simulink model "etp_model"  (R2026a)
settings: Solver=ode15s  StartTime=0  StopTime=1800  MaxStep=0.5  RelTol=1e-6  AbsTol=1e-9
InitFcn:
  | if ~evalin('base','exist(''Qext_ts'',''var'')'),
  |   p_ = evalin('base','p');
  |   Qext_ts = timeseries(p_.Qext_profile.value, p_.Qext_profile.time);
  |   assignin('base','Qext_ts',Qext_ts);
  | end
settings Model: Creator=fsk  LastModifiedBy=fsk

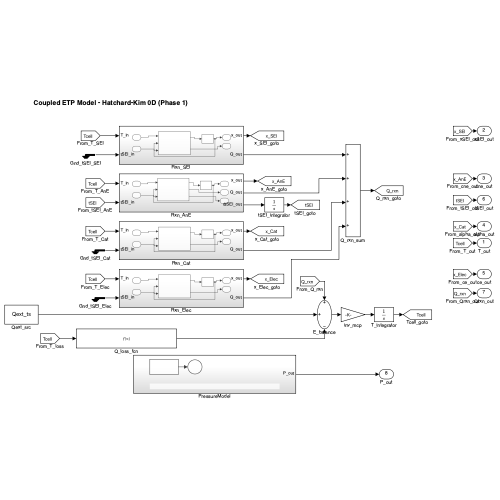
[thumbnail: Simulink's stored preview of the top-level diagram]
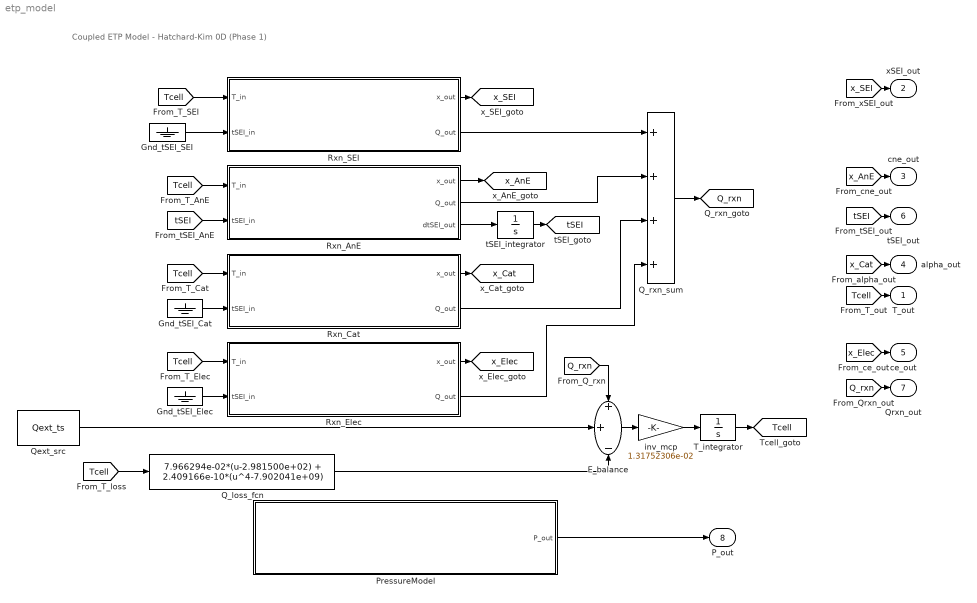
== system etp_model ==
  note: Coupled ETP Model - Hatchard-Kim 0D (Phase 1)
  E_balance : Sum  Inputs=++-
  Gnd_tSEI_Cat : Ground
  Gnd_tSEI_Elec : Ground
  Gnd_tSEI_SEI : Ground
  PressureModel : Subsystem
  Q_loss_fcn : Fcn  Expr=7.966294e-02*(u-2.981500e+02) + 2.409166e-10*(u^4-7.902041e+09)
  Q_rxn_sum : Sum  Inputs=++++
  Qext_src : FromWorkspace  VariableName=Qext_ts  OutputAfterFinalValue=Holding final value
  Rxn_AnE : Subsystem
  Rxn_Cat : Subsystem
  Rxn_Elec : Subsystem
  Rxn_SEI : Subsystem
  T_integrator : Integrator  InitialCondition=298.150000
  inv_mcp : Gain  Gain=1.31752306e-02
  tSEI_integrator : Integrator  InitialCondition=3.30000000e-02
  T_out : Outport
  xSEI_out : Outport  Port=2
  cne_out : Outport  Port=3
  alpha_out : Outport  Port=4
  ce_out : Outport  Port=5
  tSEI_out : Outport  Port=6
  Qrxn_out : Outport  Port=7
  P_out : Outport  Port=8
  tag scope: Q_rxn=global, Tcell=global, tSEI=global, x_AnE=global, x_Cat=global, x_Elec=global, x_SEI=global
  wires:
  [Tcell] -> Q_loss_fcn/1
  [Tcell] -> Rxn_SEI/1(T_in)
  Gnd_tSEI_SEI/1 -> Rxn_SEI/2(tSEI_in)
  Rxn_SEI/1(x_out) -> [x_SEI]
  [Tcell] -> Rxn_AnE/1(T_in)
  [tSEI] -> Rxn_AnE/2(tSEI_in)
  Rxn_AnE/1(x_out) -> [x_AnE]
  [Tcell] -> Rxn_Cat/1(T_in)
  Gnd_tSEI_Cat/1 -> Rxn_Cat/2(tSEI_in)
  Rxn_Cat/1(x_out) -> [x_Cat]
  [Tcell] -> Rxn_Elec/1(T_in)
  Gnd_tSEI_Elec/1 -> Rxn_Elec/2(tSEI_in)
  Rxn_Elec/1(x_out) -> [x_Elec]
  Rxn_SEI/2(Q_out) -> Q_rxn_sum/1
  Rxn_AnE/2(Q_out) -> Q_rxn_sum/2
  Rxn_Cat/2(Q_out) -> Q_rxn_sum/3
  Rxn_Elec/2(Q_out) -> Q_rxn_sum/4
  Q_rxn_sum/1 -> [Q_rxn]
  [Q_rxn] -> E_balance/1
  Qext_src/1 -> E_balance/2
  Q_loss_fcn/1 -> E_balance/3
  E_balance/1 -> inv_mcp/1
  inv_mcp/1 -> T_integrator/1
  T_integrator/1 -> [Tcell]
  Rxn_AnE/3(dtSEI_out) -> tSEI_integrator/1
  tSEI_integrator/1 -> [tSEI]
  [Tcell] -> T_out/1
  [x_SEI] -> xSEI_out/1
  [x_AnE] -> cne_out/1
  [x_Cat] -> alpha_out/1
  [x_Elec] -> ce_out/1
  [tSEI] -> tSEI_out/1
  [Q_rxn] -> Qrxn_out/1
  PressureModel/1(P_out) -> P_out/1

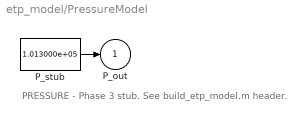
== system etp_model/PressureModel ==
  note: PRESSURE - Phase 3 stub. See build_etp_model.m header.
  P_stub : Constant  Value=1.013000e+05
  P_out : Outport
  wires:
  P_stub/1 -> P_out/1

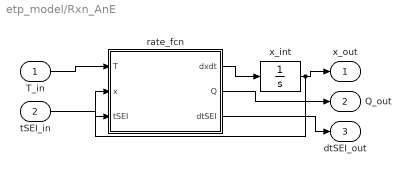
== system etp_model/Rxn_AnE ==
  T_in : Inport
  tSEI_in : Inport  Port=2
  rate_fcn : MATLAB Function  TreatAsAtomicUnit=on
  x_int : Integrator  InitialCondition=7.50000000e-01
  x_out : Outport
  Q_out : Outport  Port=2
  dtSEI_out : Outport  Port=3
  wires:
  T_in/1 -> rate_fcn/1(T)
  x_int/1 -> rate_fcn/2(x), x_out/1
  tSEI_in/1 -> rate_fcn/3(tSEI)
  rate_fcn/1(dxdt) -> x_int/1
  rate_fcn/2(Q) -> Q_out/1
  rate_fcn/3(dtSEI) -> dtSEI_out/1

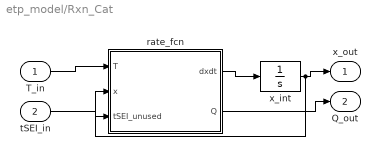
== system etp_model/Rxn_Cat ==
  T_in : Inport
  tSEI_in : Inport  Port=2
  rate_fcn : MATLAB Function  TreatAsAtomicUnit=on
  x_int : Integrator  InitialCondition=4.00000000e-02
  x_out : Outport
  Q_out : Outport  Port=2
  wires:
  T_in/1 -> rate_fcn/1(T)
  x_int/1 -> rate_fcn/2(x), x_out/1
  tSEI_in/1 -> rate_fcn/3(tSEI_unused)
  rate_fcn/1(dxdt) -> x_int/1
  rate_fcn/2(Q) -> Q_out/1

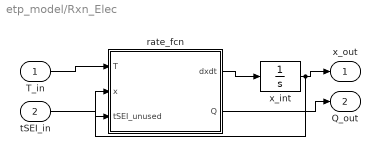
== system etp_model/Rxn_Elec ==
  T_in : Inport
  tSEI_in : Inport  Port=2
  rate_fcn : MATLAB Function  TreatAsAtomicUnit=on
  x_int : Integrator  InitialCondition=1.00000000e+00
  x_out : Outport
  Q_out : Outport  Port=2
  wires:
  T_in/1 -> rate_fcn/1(T)
  x_int/1 -> rate_fcn/2(x), x_out/1
  tSEI_in/1 -> rate_fcn/3(tSEI_unused)
  rate_fcn/1(dxdt) -> x_int/1
  rate_fcn/2(Q) -> Q_out/1

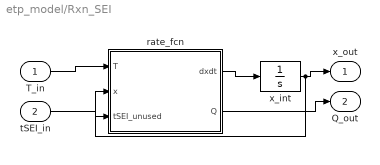
== system etp_model/Rxn_SEI ==
  T_in : Inport
  tSEI_in : Inport  Port=2
  rate_fcn : MATLAB Function  TreatAsAtomicUnit=on
  x_int : Integrator  InitialCondition=1.50000000e-01
  x_out : Outport
  Q_out : Outport  Port=2
  wires:
  T_in/1 -> rate_fcn/1(T)
  x_int/1 -> rate_fcn/2(x), x_out/1
  tSEI_in/1 -> rate_fcn/3(tSEI_unused)
  rate_fcn/1(dxdt) -> x_int/1
  rate_fcn/2(Q) -> Q_out/1

== matlab function etp_model/Rxn_AnE/rate_fcn ==
  data: T input; dxdt output; x input; tSEI input; Q output; dtSEI output
function [dxdt, Q, dtSEI] = rate_fcn(T, x, tSEI)
%#codegen
A     = 2.50000000e+13;
Ea    = 1.35080000e+05;
dH    = 1.71400000e+06;
w     = 6.10400000e+02;
V     = 2.42452413e-05;
Ru    = 8.31400000e+00;
c     = -1;
tSEI0 = 3.30000000e-02;
g     = exp(-tSEI/tSEI0);
R     = A * exp(-Ea/(Ru*T)) * max(x,0) * g;
dxdt  = c * R;
Q     = w * V * dH * R;
dtSEI = R;
end

== matlab function etp_model/Rxn_SEI/rate_fcn ==
  data: T input; dxdt output; x input; tSEI_unused input; Q output
function [dxdt, Q] = rate_fcn(T, x, tSEI_unused)
%#codegen
A    = 1.66700000e+15;
Ea   = 1.35080000e+05;
dH   = 2.57000000e+05;
w    = 6.10400000e+02;
V    = 2.42452413e-05;
Ru   = 8.31400000e+00;
c    = -1;
R = A * exp(-Ea/(Ru*T)) * max(x,0);
dxdt = c * R;
Q    = w * V * dH * R;
end

== matlab function etp_model/Rxn_Cat/rate_fcn ==
  data: T input; dxdt output; x input; tSEI_unused input; Q output
function [dxdt, Q] = rate_fcn(T, x, tSEI_unused)
%#codegen
A    = 6.66700000e+13;
Ea   = 1.39600000e+05;
dH   = 3.14000000e+05;
w    = 1.22100000e+03;
V    = 2.42452413e-05;
Ru   = 8.31400000e+00;
c    = 1;
R = A * exp(-Ea/(Ru*T)) * max(x,0) * max(1-x,0);
dxdt = c * R;
Q    = w * V * dH * R;
end

== matlab function etp_model/Rxn_Elec/rate_fcn ==
  data: T input; dxdt output; x input; tSEI_unused input; Q output
function [dxdt, Q] = rate_fcn(T, x, tSEI_unused)
%#codegen
A    = 5.14000000e+25;
Ea   = 2.74000000e+05;
dH   = 1.55000000e+05;
w    = 4.06900000e+02;
V    = 2.42452413e-05;
Ru   = 8.31400000e+00;
c    = -1;
R = A * exp(-Ea/(Ru*T)) * max(x,0);
dxdt = c * R;
Q    = w * V * dH * R;
end
